simulink model "simXplane"  (R2020a)
settings: Solver=VariableStepAuto  StartTime=0.0  StopTime=inf  RelTol=1e-3
libraries: etargetslib x1, dspnetwork x1
settings Model: Creator=don  LastModifiedBy=don

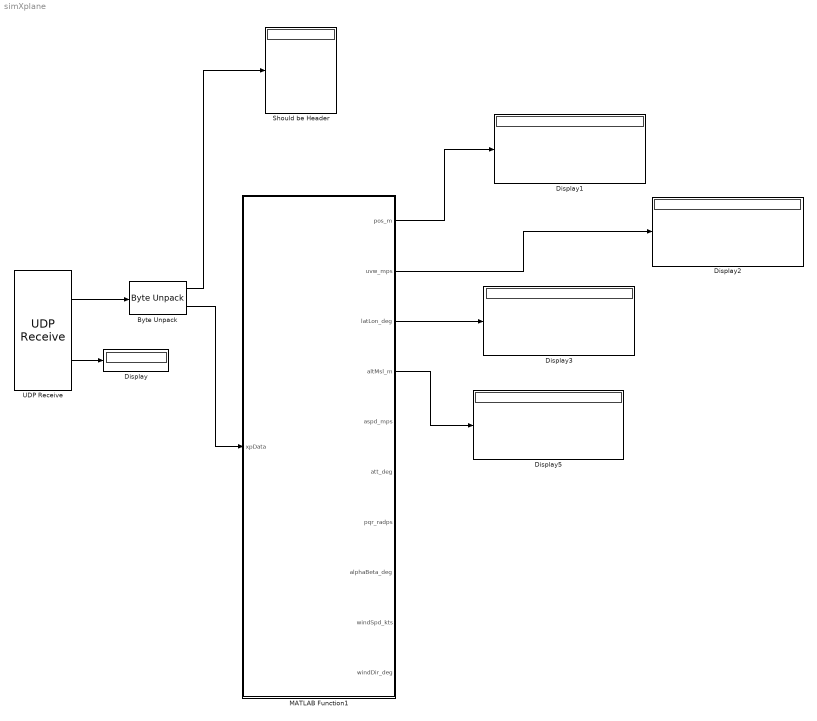
== system simXplane ==
  Byte Unpack : etargetslib/Byte Unpack  dimensions={5,[9,16]}  datatypes={'uint8','single'}  byteAlign=1
  Display{,1..3,5} (5 alike) : Display
  MATLAB Function1 : MATLAB Function  TreatAsAtomicUnit=on
  Should be Header : Display
  UDP Receive : dspnetwork/UDP Receive  localURL='0.0.0.0'  localPort=49004  remoteURL='127.0.0.1'  remotePort=-1  recvBufferSize=8192  dims=(5 + 16*9*4)  signalDatatype=uint8  isComplex=off  isVarSize=off  showBlockingTime=off  blockingTime=0  sampletime=inf  blockPlatform=[]
  wires:
  Byte Unpack/1 -> Should be Header/1
  UDP Receive/1 -> Byte Unpack/1
  Byte Unpack/2 -> MATLAB Function1/1(xpData)
  UDP Receive/2 -> Display/1
  MATLAB Function1/1(pos_m) -> Display1/1
  MATLAB Function1/2(uvw_mps) -> Display2/1
  MATLAB Function1/3(latLon_deg) -> Display3/1
  MATLAB Function1/4(altMsl_m) -> Display5/1

== matlab function simXplane/MATLAB Function1 ==
  data: xpData input; pos_m output; uvw_mps output; latLon_deg output; altMsl_m output; aspd_mps output; att_deg output; pqr_radps output; alphaBeta_deg output; windSpd_kts output; windDir_deg output
function [pos_m, uvw_mps, latLon_deg, altMsl_m, aspd_mps, att_deg, pqr_radps, alphaBeta_deg, windSpd_kts, windDir_deg] = fcn(xpData)

% The order of the data output depends on the order at which XP outputs
ft2m = 0.3048;
ftlb2Nm = 1.36;
kts2mps = 0.514444;

speedsData          = xpData(:, 1);
machData            = xpData(:, 2);
weatherData         = xpData(:, 3);
atmosData           = xpData(:, 4);
joystickData        = xpData(:, 5);
fcData              = xpData(:, 6);
angularMomentsData  = xpData(:, 7);
angularVelocityData = xpData(:, 8);
attitudeData        = xpData(:, 9);
aoaData             = xpData(:, 10);
llaData             = xpData(:, 11);
localPosVelData     = xpData(:, 12);
thrCmdData          = xpData(:, 13);
thrActualData       = xpData(:, 14);
engineThrustData    = xpData(:, 15);
propRpmData         = xpData(:, 16);

% Airspeed
aspdTrue_kts = speedsData(5); % "True airspeed, in knots true ground speed"
aspd_mps = aspdTrue_kts * kts2mps;

% Loads
machNumber_mach = machData(2);
verticalVelInertial = machData(3);
loadNormal_g = machData(6);
loadAxial_g = machData(7);
loadSide_g = machData(8);
bodyLoads_g = [loadAxial_g, loadSide_g, loadNormal_g];

% Weather
windSpd_kts = weatherData(4);
windDir_deg = weatherData(5);

% Atmosphere
dynPressure = atmosData(7);

% Joystick 
elevStick_perc = joystickData(2);
ailStick_perc = joystickData(3);
rudStick_perc = joystickData(4);

% angularMomentsData
L_ftlb = angularMomentsData(2);
M_ftlb = angularMomentsData(3);
N_ftlb = angularMomentsData(4);
LMN_Nm = [L_ftlb, M_ftlb, N_ftlb]*ftlb2Nm;

% angularVelocityData
p_radps = angularVelocityData(2);
q_radps = angularVelocityData(3);
r_radps = angularVelocityData(4);
pqr_radps = [p_radps, q_radps, r_radps];

% Attitude 
theta_deg = attitudeData(2);
phi_deg = attitudeData(3);
psi_deg = attitudeData(4);
att_deg = [theta_deg, phi_deg, psi_deg];

% AoA data
alpha_deg = aoaData(2);
beta_deg = aoaData(3);
hpath_deg = aoaData(4);
vpath_deg = aoaData(5);

alphaBeta_deg = [alpha_deg, beta_deg];

% Flight path
gamma_deg = aoaData(5);

% LLA
lat_deg = llaData(2);
lon_deg = llaData(3);
altMsl_ft = llaData(4);
altAgl_ft = llaData(5);
latLon_deg = [lat_deg, lon_deg];
altMsl_m = altMsl_ft * ft2m;

% localPosVelData
posX_m = localPosVelData(2);
posY_m = localPosVelData(3);
posZ_m = localPosVelData(4);
pos_m = [posX_m, posY_m, posZ_m];

u_mps = localPosVelData(5);
v_mps = localPosVelData(6);
w_mps = localPosVelData(7);
uvw_mps = [u_mps, v_mps, w_mps];

% Throttles
thrCmd_perc = thrCmdData(2);
thrActual_perc = thrActualData(2);

% Propeller
propRpm_rpm = propRpmData(2);


end
